simulink model "RobotX_ss_acousticsSingle_Dock_LB_ODOA_1024"  (R2014a)
settings: Solver=FixedStepDiscrete  StartTime=0.0  StopTime=inf  FixedStep=.25  RelTol=1e-3
undefined symbols (not defined in the file): Com1, Com2, Com3, Com4, DiscIntNeverNeededParam, standard
libraries: xpcseriallib x42, simulink x19, slrtlib x7, dspmtrx3 x2, speedgoatlib x2, speedgoatlib_IO102 x1
(part 6 of 7)

== matlab function RobotX_ss_acousticsSingle_Dock_LB_ODOA_1024/Sensors/1024 Comms/Message Selector/HRT Message/MATLAB Function ==
  data: Time input; asciiHRT output; HRTLat input; HRTLong input; HRTMode input; HRTTask input
% This function creates the heartbeat message to be sent from Speedgoat in
% ascii code
% Written by: Edward Zhu
% Date: 9/17/14

function asciiHRT = asciiHRTEncoder(Time, HRTLat, HRTLong, HRTMode, HRTTask)

% Initialize output message vector as the serial output block expects 128
% character message
asciiHRT = uint8(zeros(1,128));

% Convert static strings to ascii code
asciiHRTMsgID = uint8('$RXHRT,');
asciiComma = uint8(',');
asciiDeciPt = uint8('.');
if HRTLat >= 0
    asciiHRTNS = uint8('N,');
else
    HRTLat = -HRTLat;
    asciiHRTNS = uint8('S,');
end
if HRTLong >= 0
    asciiHRTEW = uint8('E,');
else
    HRTLong = -HRTLong;
    asciiHRTEW = uint8('W,');
end
asciiTeamID = uint8('FAUVU,');
asciiMsgEnd = uint8('*');
asciiMsgCRLF = [13 10];

% Convert UTC Time input (hhmmss) into ascii code
asciiTime = uint8(zeros(1,7));
asciiTime(7) = asciiComma;

for timeChar = 1:6
    asciiTime(timeChar) = floor(mod(Time,10^(7-timeChar))/...
        10^(6-timeChar)) + 48;
end

% Convert latitude (dd.mmmmmm) into ascii code
asciiHRTLat = uint8(zeros(1,10));
asciiHRTLat(10) = asciiComma;
asciiHRTLat(3) = asciiDeciPt;

HRTlatInt = floor(HRTLat);
for latIntChar = 1:2
    asciiHRTLat(latIntChar) = floor(mod(HRTlatInt,10^(3-latIntChar))/...
        10^(2-latIntChar)) + 48;
end

HRTlatDeci = mod(HRTLat,HRTlatInt) * 10^6;
for latDeciChar = 1:6
    asciiHRTLat(latDeciChar+3) = floor(mod(HRTlatDeci,10^(7-latDeciChar))/...
        10^(6-latDeciChar)) + 48;
end

% Convert longitude (ddd.mmmmmm) into ascii code
asciiHRTLong = uint8(zeros(1,11));
asciiHRTLong(11) = asciiComma;
asciiHRTLong(4) = asciiDeciPt;

HRTlongInt = floor(HRTLong);
for longIntChar = 1:3
    asciiHRTLong(longIntChar) = floor(mod(HRTlongInt,10^(4-longIntChar))/...
        10^(3-longIntChar)) + 48;
end

HRTlongDeci = mod(HRTLong,HRTlongInt) * 10^6;
for longDeciChar = 1:6
    asciiHRTLong(longDeciChar+4) = floor(mod(HRTlongDeci,10^(7-longDeciChar))/...
        10^(6-longDeciChar)) + 48;
end


% Convert vehicle mode into ascii (1 = RC, 2 = Auto)

% Auto On 
if HRTMode == 3 
    HRTOpMode = 2;
    asciiHRTMode = [uint8(HRTOpMode+48) asciiComma];
else
    HRTOpMode = 1;
    asciiHRTMode = [uint8(HRTOpMode+48) asciiComma];
end

% Convert vehicle task into ascii
HRTTask = HRTTask - 1; % FSM: Init = 1, SSGate = 2, SEA = 3, Dock = 4, LIT = 5, Obst = 6
if HRTTask ~= 1 || 2 || 3 || 4 || 5
    HRTOpTask = 1;
    asciiHRTTask = [uint8(HRTOpTask+48) asciiMsgEnd];
else
    asciiHRTTask = [uint8(HRTTask+48) asciiMsgEnd];
end

% Concat individual ascii arrays into one array
asciiHRTPreChkSum = cat(2,asciiHRTMsgID,asciiTime,asciiHRTLat,asciiHRTNS,asciiHRTLong,asciiHRTEW,...
    asciiTeamID,asciiHRTMode,asciiHRTTask);

% Calculate the checksum of the message from the '$' to the '*' and convert
% to hex
HRTchkSum = uint8(0);

for chksumChar = 1:(length(asciiHRTPreChkSum)-2)
    HRTchkSum = bitxor(HRTchkSum,asciiHRTPreChkSum(chksumChar+1));
end

% Convert the checksum to ascii
HRTchkSum = dec2hex(HRTchkSum);
asciiHRTChkSum = uint8(zeros(1,length(HRTchkSum))+32);
for i = 1:length(HRTchkSum)
    asciiHRTChkSum(i) = uint8(HRTchkSum(i));
end

% Concat the checksum and the '/r/n' to the end of the message
asciiHRTPostChkSum = cat(2,asciiHRTPreChkSum,asciiHRTChkSum,asciiMsgCRLF);

% Output the final message
asciiHRT(1:length(asciiHRTPostChkSum)) = asciiHRTPostChkSum;

== matlab function RobotX_ss_acousticsSingle_Dock_LB_ODOA_1024/Sensors/1024 Comms/Message Selector/HRTLIT Message/MATLAB Function ==
  data: Time input; HRTLat input; HRTLong input; HRTTask input; HRTMode input; LITValid input; asciiHRTLIT output; LITSequence input
function asciiHRTLIT = asciiHRTLITEncoder(Time,HRTLat,HRTLong,HRTTask,HRTMode,LITValid,LITSequence)
% Initialize output message vector as the serial output block expects 128
% character message
asciiHRTLIT = uint8(zeros(1,128));

asciiComma = uint8(',');
asciiDeciPt = uint8('.');
asciiTeamID = uint8('FAUVU,');
asciiMsgEnd = uint8('*');
asciiMsgCRLF = [13 10];

% Convert UTC Time input (hhmmss) into ascii code
asciiTime = uint8(zeros(1,7));
asciiTime(7) = asciiComma;

for timeChar = 1:6
    asciiTime(timeChar) = floor(mod(Time,10^(7-timeChar))/...
        10^(6-timeChar)) + 48;
end

%%%%%%%%%%%%%%%%%%%%%%%%%%%%%%%%%%%%%%%%%%%%%%%%%%%%%%%%%%%%%%%%%%%%
% Heartbeat message
% Convert static strings to ascii code
asciiHRTMsgID = uint8('$RXHRT,');
if HRTLat >= 0
    asciiHRTNS = uint8('N,');
else
    HRTLat = -HRTLat;
    asciiHRTNS = uint8('S,');
end
if HRTLong >= 0
    asciiHRTEW = uint8('E,');
else
    HRTLong = -HRTLong;
    asciiHRTEW = uint8('W,');
end

% Convert latitude (dd.mmmmmm) into ascii code
asciiHRTLat = uint8(zeros(1,10));
asciiHRTLat(10) = asciiComma;
asciiHRTLat(3) = asciiDeciPt;

HRTlatInt = floor(HRTLat);
for latIntChar = 1:2
    asciiHRTLat(latIntChar) = floor(mod(HRTlatInt,10^(3-latIntChar))/...
        10^(2-latIntChar)) + 48;
end

HRTlatDeci = mod(HRTLat,HRTlatInt) * 10^6;
for latDeciChar = 1:6
    asciiHRTLat(latDeciChar+3) = floor(mod(HRTlatDeci,10^(7-latDeciChar))/...
        10^(6-latDeciChar)) + 48;
end

% Convert longitude (ddd.mmmmmm) into ascii code
asciiHRTLong = uint8(zeros(1,11));
asciiHRTLong(11) = asciiComma;
asciiHRTLong(4) = asciiDeciPt;

HRTlongInt = floor(HRTLong);
for longIntChar = 1:3
    asciiHRTLong(longIntChar) = floor(mod(HRTlongInt,10^(4-longIntChar))/...
        10^(3-longIntChar)) + 48;
end

HRTlongDeci = mod(HRTLong,HRTlongInt) * 10^6;
for longDeciChar = 1:6
    asciiHRTLong(longDeciChar+4) = floor(mod(HRTlongDeci,10^(7-longDeciChar))/...
        10^(6-longDeciChar)) + 48;
end

% Convert vehicle mode into ascii (1 = RC, 2 = Auto)

% Auto On 
if HRTMode == 3 
    HRTOpMode = 2;
    asciiHRTMode = [uint8(HRTOpMode+48) asciiComma];
else
    HRTOpMode = 1;
    asciiHRTMode = [uint8(HRTOpMode+48) asciiComma];
end

% Convert vehicle task into ascii
HRTTask = HRTTask - 1; % FSM: Init = 1, SSGate = 2, SEA = 3, Dock = 4, LIT = 5, Obst = 6
if HRTTask ~= 1 || 2 || 3 || 4 || 5
    HRTOpTask = 1;
    asciiHRTTask = [uint8(HRTOpTask+48) asciiMsgEnd];
else
    asciiHRTTask = [uint8(HRTTask+48) asciiMsgEnd];
end

% Concat individual ascii arrays into one array
asciiHRTPreChkSum = cat(2,asciiHRTMsgID,asciiTime,asciiHRTLat,asciiHRTNS,asciiHRTLong,asciiHRTEW,...
    asciiTeamID,asciiHRTMode,asciiHRTTask);

% Calculate the checksum of the message from the '$' to the '*' and convert
% to hex
HRTchkSum = uint8(0);

for chksumChar = 1:(length(asciiHRTPreChkSum)-2)
    HRTchkSum = bitxor(HRTchkSum,asciiHRTPreChkSum(chksumChar+1));
end

% Convert the checksum to ascii
HRTchkSum = dec2hex(HRTchkSum);
asciiHRTChkSum = uint8(zeros(1,length(HRTchkSum))+32);
for i = 1:length(HRTchkSum)
    asciiHRTChkSum(i) = uint8(HRTchkSum(i));
end

% Concat the checksum and the '/r/n' to the end of the message
asciiHRTPostChkSum = cat(2,asciiHRTPreChkSum,asciiHRTChkSum,asciiMsgCRLF);

%%%%%%%%%%%%%%%%%%%%%%%%%%%%%%%%%%%%%%%%%%%%%%%%%%%%%%%%%%%%%%%%%%%%%

% Light tower message
asciiLITMsgID = uint8('$RXLIT,');

% Convert the light sequece into ascii code (1 = R, 2 = B, 3 = G)
asciiLITSeq = uint8(zeros(1,4)+32);
asciiLITSeq(4) = asciiMsgEnd;

if LITValid == 1
    for seqChar = 1:3
        if LITSequence(seqChar) == 1
            LITSequence(seqChar) = uint8('R');
        elseif LITSequence(seqChar) == 2
            LITSequence(seqChar) = uint8('B');
        elseif LITSequence(seqChar) == 3
            LITSequence(seqChar) = uint8('G');
        end
    end
    asciiLITSeq(1:3) = LITSequence;
end

% Concat individual ascii arrays into one array
asciiLITPreChkSum = cat(2,asciiLITMsgID,asciiTime,asciiTeamID,asciiLITSeq);

% Calculate the checksum of the message from the '$' to the '*' and convert
% to hex
LITchkSum = uint8(0);

for chksumChar = 1:(length(asciiLITPreChkSum)-2)
    LITchkSum = bitxor(LITchkSum,asciiLITPreChkSum(chksumChar+1));
end

% Convert the checksum to ascii
LITchkSum = dec2hex(LITchkSum);
asciiLITChkSum = uint8(zeros(1,length(LITchkSum))+32);
for i = 1:length(LITchkSum)
    asciiLITChkSum(i) = uint8(LITchkSum(i));
end

% Concat the checksum and the '/r/n' to the end of the message
asciiLITPostChkSum = cat(2,asciiLITPreChkSum,asciiLITChkSum,asciiMsgCRLF);

%%%%%%%%%%%%%%%%%%%%%%%%%%%%%%%%%%%%%%%%%%%%%%%%%%%%%%%%%%%%%%%%%%%%%%%%%%%

asciiHRTLITPostChkSum = cat(2,asciiHRTPostChkSum,asciiLITPostChkSum);
asciiHRTLIT(1:length(asciiHRTLITPostChkSum)) = asciiHRTLITPostChkSum;

== matlab function RobotX_ss_acousticsSingle_Dock_LB_ODOA_1024/Main FSM/Acoustic Single Point FSM/Report/MATLAB Function ==
  data: X input; Y input; Psi input; Data output
function Data  = Orient(X, Y, Psi)
%Written by Dylan DeGaetano on September 2, 2014
%Last Edited:Dylan DeGaetano on September 10,2014

%This function passes the current pose data added to the angle of the Light 
%buoy This stare forces the Boat to stare at the bouy.This task must be in station 
%keeping mode

persistent holdPose

if isempty(holdPose)
    holdPose = [X, Y, Psi];
end

%Initialize Data variable
Data = zeros(24,1);

%Set desired pose
Data(1) = holdPose(1);
Data(2) = holdPose(2);
Data(3) = holdPose(3);

end

== matlab function RobotX_ss_acousticsSingle_Dock_LB_ODOA_1024/Main FSM/Start//Speedgate/Aim/LLA to NED ==
  data: LLA input; GoalNED output; NED_origin input
function GoalNED = LLA2NEDfun(LLA,NED_origin)
%Written by Anderson Lebbad on September 20, 2014
%Last edited by:
%
%This function converts a target Latitude, Longitude, Altitude (LLA) point
%into North, East, Down (NED) coordinates

%First convert to earth centered, earth fixed frame
GoalECEF = lla2ecef([LLA*(pi/180), 0]');
%Then convert from ECEF to North East Down
GoalNEDvect = ecef2ned(NED_origin'*(pi/180),GoalECEF);
GoalNED = GoalNEDvect(1:2)';


end

function x_ecef = lla2ecef(x_lla)
% LLE2ECEF: Converts from geodetic latitude, longitude, and altitude to earth-centered earth-fixed Cartesian coordinates
% INPUT: latitude phi (rad), longitude lambda (rad), altitude h (m)
% OUTPUT: [x, y, z]' (m) earth-centered earth-fixed Cartesian coordinates
    a = 6378137; % equatorial radius of ellipsoid (semi-major axis) (m)
    b = 6356752; % polar axis radius of ellipsoid (semi-minor axis) (m)

    phi = x_lla(1);
    lambda = x_lla(2);
    h = x_lla(3);
    
    % auxiliar quantities f, e, and N
    f = (a-b)/a;
    e = f*(2-f);
    N = a/sqrt(1-(e*sin(phi))^2);
    x_ecef = [(N+h)*cos(phi)*cos(lambda); (N+h)*cos(phi)*sin(lambda); (N*(1-e^2)+h)*sin(phi)];
end

function [x_ned] = ecef2ned(ned_lla, x_ecef)
% ECEF2NED Converts from earth-centered, earth-fixed Cartesian coordinates to tangent plane
% INPUT:
% 1) x_ecef=[x,y,z]' (m) earth-centered, earth-fixed Cartesian coordinates
% 2) ned_lla=[phi,lambda]' consiting of latitude phi (rad), longitude lambda (rad) of NED origin
% OUTPUT:
% 1) x_ned=[x,y,z]' (m) in NED coordinate system with the origin [phi,lambda]'

    phi = ned_lla(1);
    lambda = ned_lla(2);

    % transformation  matrix
    T = [-sin(phi)*cos(lambda) -sin(phi)*sin(lambda)  cos(phi)
         -sin(lambda)           cos(lambda)           0
          cos(phi)*cos(lambda)   cos(phi)*sin(lambda)  sin(phi)];

     x_ned = T*(x_ecef-lla2ecef([phi, lambda, 0]')); % convert to NED
     x_ned(3) = -x_ned(3);
end

== matlab function RobotX_ss_acousticsSingle_Dock_LB_ODOA_1024/Main FSM/LightTower/Approach Light Tower/GPSMove ==
  data: GoalNED input; X input; Finished output; valid output; Y input; Psi input; pts output
function [Finished,valid,pts] = GPSmove(GoalNED,X,Y,Psi)
%Written by Dylan DeGaetano on September 1, 2014
%Last edited by: Anderson Lebbad
%
%This function will go to a given NED cooridnate, last edit changed the
%goal pt and variable names

persistent Sample
if isempty(Sample)
Sample = 0;
end
Finished = 0;
pts = zeros(8,2);

%If this has been going for a while, reset.
if Sample == 100
    Sample = 0;
end

%If we need to calculate desired points to send, calculate them.
if Sample == 0
    pts(1,1) = X+5*cos(Psi*pi/180);
    pts(1,2) = Y+5*sin(Psi*pi/180);
    pts(8,1) = GoalNED(1,1);
    pts(8,2) = GoalNED(1,2);
    pts(2,:) = pts(1,:) +(1*(GoalNED-pts(1,:))/7);
    pts(3,:) = pts(1,:) +(2*(GoalNED-pts(1,:))/7);
    pts(4,:) = pts(1,:) +(3*(GoalNED-pts(1,:))/7);
    pts(5,:) = pts(1,:) +(4*(GoalNED-pts(1,:))/7);
    pts(6,:) = pts(1,:) +(5*(GoalNED-pts(1,:))/7);
    pts(7,:) = pts(1,:) +(6*(GoalNED-pts(1,:))/7);
    Sample = 1; 
    valid = 1;
    
%If we have already calculated desired points, check if we are within a
%certain range of the desired end point.
else 
    range = sqrt(sum((GoalNED - [X Y]).^2));
    if range <= 5
        Finished = 1;
    end
    valid = 0;
    Sample = Sample + 1;
end

== matlab function RobotX_ss_acousticsSingle_Dock_LB_ODOA_1024/Main FSM/LightTower/Approach Light Tower/MATLAB Function ==
  data: HoldPose output; distance input; ltLoc input; GoalNED output; X input; Y input
function [HoldPose, GoalNED] = fcn(distance, ltLoc, X, Y)
%Written by Michael Benson on October 23, 2014

%This function determines the target NED point for the Sweep Field subtask
%for the Light Tower task.  The target point is Distance meters from the
%current ASV position, and is towards the opposite corner of the subset
%field.

%Find slope between ASV and corner
% slope = (ltLoc(2) - Y)/(ltLoc(1) - X);
% GoalNED = [X - distance*cos(slope), Y - distance*sin(slope)];

pts = zeros(1,2);
desiredHeading = atan2(ltLoc(2)-Y,ltLoc(1)-X);
pts(1,1) = ltLoc(1)+distance*cos(desiredHeading);
pts(1,2) = ltLoc(2)+distance*sin(desiredHeading);
GoalNED = [pts(1,1) pts(1,2)];

holdHeading = atan2(ltLoc(2)-GoalNED(2),ltLoc(1)-GoalNED(1))*180/pi;
HoldPose = [GoalNED, holdHeading];

end

== matlab function RobotX_ss_acousticsSingle_Dock_LB_ODOA_1024/Main FSM/LightTower/Go to Field Corner/CalcTimes ==
  data: pts input; u input; Data output
function Data = calcTimes(pts, u)
%Written by Anderson Lebbad on August 9, 2014
%Last Edited: Dylan DeGaetano September 1, 2014

%Calculates times for the boat to get to points for a trajectory, and
%formats Data for communication

%Initialize
Data = zeros(24,1);
traj = zeros(8,3);
traj(:,1:2) = pts;



for k = 2:8
    %Calculate distance to travel from last point
    distTravel = sqrt(sum((pts(k-1,:)-pts(k,:)).^2));
    %Assume 1m per second speed
    traj(k,3) = traj(k-1,3) + distTravel;
    %Add time based off initial velocity to get to first point past initial
    if k == 2
        traj(k,3) = traj(k,3) + 2.5*abs(2-u);
    end
end


%Output Data
for i=1:8
    for j = 1:3
        Data(3*(i-1)+j) = traj(i,j);
    end
end

== matlab function RobotX_ss_acousticsSingle_Dock_LB_ODOA_1024/Main FSM/Start//Speedgate/Aim/MATLAB Function ==
  data: ssHeldHeading input; ssGateNED input; Data output
function Data  = Orient(ssHeldHeading,ssGateNED)
%Written by Dylan DeGaetano on September 2, 2014
%Last Edited:Dylan DeGaetano on September 10,2014

%This function passes the current pose data added to the angle of the Light 
%buoy This stare forces the Boat to stare at the bouy.This task must be in station 
%keeping mode

persistent holdPose

if isempty(holdPose)
    holdPose = [ssGateNED ssHeldHeading];
end

%Initialize Data variable
Data = zeros(24,1);

%Set desired pose
Data(1) = holdPose(1);
Data(2) = holdPose(2);
Data(3) = holdPose(3);

end

== matlab function RobotX_ss_acousticsSingle_Dock_LB_ODOA_1024/Main FSM/LightTower/Go to Field Corner/GPSMove ==
  data: GoalNED input; X input; Finished output; valid output; Y input; Psi input; pts output
function [Finished,valid,pts] = GPSmove(GoalNED,X,Y,Psi)
%Written by Dylan DeGaetano on September 1, 2014
%Last edited by: Anderson Lebbad
%
%This function will go to a given NED cooridnate, last edit changed the
%goal pt and variable names

% Input of GoalNED is a 10x2 matrix of NED coords where the first row is
% the coord of the docking observation point

persistent Sample
if isempty(Sample)
Sample = 0;
end
Finished = 0;
pts = zeros(8,2);
%$Distance to object in meters
if Sample == 100
    Sample = 0;
end

if Sample == 0
    pts(1,1) = X+5*cos(Psi*pi/180);
    pts(1,2) = Y+5*sin(Psi*pi/180);
    pts(8,1) = GoalNED(1,1);
    pts(8,2) = GoalNED(1,2);
    pts(2,:) = pts(1,:) +(1*(GoalNED(1,:)-pts(1,:))/7);
    pts(3,:) = pts(1,:) +(2*(GoalNED(1,:)-pts(1,:))/7);
    pts(4,:) = pts(1,:) +(3*(GoalNED(1,:)-pts(1,:))/7);
    pts(5,:) = pts(1,:) +(4*(GoalNED(1,:)-pts(1,:))/7);
    pts(6,:) = pts(1,:) +(5*(GoalNED(1,:)-pts(1,:))/7);
    pts(7,:) = pts(1,:) +(6*(GoalNED(1,:)-pts(1,:))/7);
    Sample = 1; 
    valid = 1;
    
else 
    range = sqrt(sum((GoalNED(1,:) - [X Y]).^2));
    if range <= 5
        Finished = 1;
    end
    valid = 0;
    Sample = Sample + 1;
end

== matlab function RobotX_ss_acousticsSingle_Dock_LB_ODOA_1024/Main FSM/Start//Speedgate/Dead Reckon/Calculate Times ==
  data: pts input; u input; Data output
function Data = calcTimes(pts, u)
%Written by Anderson Lebbad on August 9, 2014
%Last Edited:

%Calculates times for the boat to get to points for a trajectory, and
%formats Data for communication

%Initialize
Data = zeros(24,1);
traj = zeros(8,3);

traj(:,1:2) = pts;

for k = 2:8
    %Calculate distance to travel from last point
    distTravel = sqrt(sum((pts(k-1,:)-pts(k,:)).^2));
    %Assume 1m per second speed
    traj(k,3) = traj(k-1,3) + distTravel;
    %Add time based off initial velocity to get to first point past initial
    if k == 2
        traj(k,3) = traj(k,3) + 2.5*abs(2-u);
    end
end


%Output Data
for i=1:8
    for j = 1:3
        Data(3*(i-1)+j) = traj(i,j);
    end
end

== matlab function RobotX_ss_acousticsSingle_Dock_LB_ODOA_1024/Main FSM/Start//Speedgate/Dead Reckon/Gate ==
  data: sglength input; ssHeldHeading input; Finished output; Valid output; X input; Y input; pts output
function [Finished, Valid, pts] = Gate(sglength,ssHeldHeading,X,Y)
%Written by Anderson Lebbad on August 9, 2014
%Last Edited by:

%This function sends a forward trajectory (from the initial heading read
%into it) until a landmark is found. Once the landmark is found, a
%trajectory is written to dodge around it.

pts = zeros(8,2);
Valid = 0;



persistent Found finPt
if isempty(Found)
    Found = 0;
    pts(1,1) = X + 5*cos(ssHeldHeading*pi/180);
    pts(1,2) = Y + 5*sin(ssHeldHeading*pi/180);
    pts(8,1) = X + sglength*cos(ssHeldHeading*pi/180);
    pts(8,2) = Y + sglength*sin(ssHeldHeading*pi/180);
    pts(2:7,:) = (1:6)'*(pts(8,:)-pts(1,:))/7+ones(6,1)*pts(1,:);
    Valid = 1;
    finPt = pts(8,:);
end

Finished = 0;

%Check to see how far the current pose is from the final point in the
%trajectory
range = abs(finPt(1)-X)+abs(finPt(2)-Y);


if range <= 10
    Finished = 1;
end

end

== matlab function RobotX_ss_acousticsSingle_Dock_LB_ODOA_1024/Main FSM/LightTower/Approach Light Tower/CalcTimes ==
  data: pts input; u input; Data output
function Data = calcTimes(pts, u)
%Written by Anderson Lebbad on August 9, 2014
%Last Edited: Dylan DeGaetano September 1, 2014

%Calculates times for the boat to get to points for a trajectory, and
%formats Data for communication

%Initialize
Data = zeros(24,1);
traj = zeros(8,3);
traj(:,1:2) = pts;



for k = 2:8
    %Calculate distance to travel from last point
    distTravel = sqrt(sum((pts(k-1,:)-pts(k,:)).^2));
    %Assume 1m per second speed
    traj(k,3) = traj(k-1,3) + distTravel;
    %Add time based off initial velocity to get to first point past initial
    if k == 2
        traj(k,3) = traj(k,3) + 2.5*abs(2-u);
    end
end


%Output Data
for i=1:8
    for j = 1:3
        Data(3*(i-1)+j) = traj(i,j);
    end
end

== matlab function RobotX_ss_acousticsSingle_Dock_LB_ODOA_1024/Main FSM/Main Enabler ==
  data: taskSelector output; initEn output; startgateEn output; acouEn output; dockEn output; LTEn output; ODOAEn output; termEn output; RCEn output; OnOffRCAuto input; initFin input; startgateFin input; acouFin input; dockFin input; LTFin input; ODOAFin input
function [taskSelector,initEn,startgateEn,acouEn,dockEn,LTEn,ODOAEn,termEn,RCEn] ...
    = taskEnabler(OnOffRCAuto,initFin,startgateFin,acouFin,dockFin,LTFin,ODOAFin)
%Written by Anderson Lebbad on September 13, 2014
%Last Edited by:

%Changes the value of MainMode and the enablers for the tasks within the
%Main FSM.

% Initialize enable signals
RCEn = 0;
initEn = 0;
startgateEn = 0;
termEn = 0;
acouEn = 0;
dockEn = 0;
LTEn = 0;
ODOAEn = 0;

% Set enable signals based on state completion
if initFin == 0
    initEn = 1;
    taskSelector = 1;
elseif OnOffRCAuto ~= 3
    RCEn = 1;
    taskSelector = 8;
elseif startgateFin == 0
    startgateEn = 1;
    taskSelector = 2;
elseif acouFin == 0
    acouEn = 1;
    taskSelector = 3;
elseif dockFin == 0
    dockEn = 1;
    taskSelector = 4;
elseif LTFin == 0
    LTEn = 1;
    taskSelector = 5;
elseif ODOAFin == 0
    ODOAEn = 1;
    taskSelector = 6;
else
    termEn = 1;
    taskSelector = 7;
end

== matlab function RobotX_ss_acousticsSingle_Dock_LB_ODOA_1024/Sensors/1024 Comms/Message Selector/HRTSEA Message/MATLAB Function ==
  data: Time input; HRTLat input; HRTLong input; HRTTask input; HRTMode input; SEAValid input; asciiHRTSEA output; SEALat input; SEALong input; SEAColor input; SEADepth input
function asciiHRTSEA = asciiHRTSEAEncoder(Time,HRTLat,HRTLong,HRTTask,HRTMode,SEAValid,SEALat,SEALong,SEAColor,SEADepth)

% Initialize output message vector as the serial output block expects 128
% character message
asciiHRTSEA = uint8(zeros(1,128));

asciiComma = uint8(',');
asciiDeciPt = uint8('.');
asciiTeamID = uint8('FAUVU,');
asciiMsgEnd = uint8('*');
asciiMsgCRLF = [13 10];

% Convert UTC Time input (hhmmss) into ascii code
asciiTime = uint8(zeros(1,7));
asciiTime(7) = asciiComma;

for timeChar = 1:6
    asciiTime(timeChar) = floor(mod(Time,10^(7-timeChar))/...
        10^(6-timeChar)) + 48;
end

%%%%%%%%%%%%%%%%%%%%%%%%%%%%%%%%%%%%%%%%%%%%%%%%%%%%%%%%%%%%%%%%%%%%
% Heartbeat message
% Convert static strings to ascii code
asciiHRTMsgID = uint8('$RXHRT,');
if HRTLat >= 0
    asciiHRTNS = uint8('N,');
else
    HRTLat = -HRTLat;
    asciiHRTNS = uint8('S,');
end
if HRTLong >= 0
    asciiHRTEW = uint8('E,');
else
    HRTLong = -HRTLong;
    asciiHRTEW = uint8('W,');
end

% Convert latitude (dd.mmmmmm) into ascii code
asciiHRTLat = uint8(zeros(1,10));
asciiHRTLat(10) = asciiComma;
asciiHRTLat(3) = asciiDeciPt;

HRTlatInt = floor(HRTLat);
for latIntChar = 1:2
    asciiHRTLat(latIntChar) = floor(mod(HRTlatInt,10^(3-latIntChar))/...
        10^(2-latIntChar)) + 48;
end

HRTlatDeci = mod(HRTLat,HRTlatInt) * 10^6;
for latDeciChar = 1:6
    asciiHRTLat(latDeciChar+3) = floor(mod(HRTlatDeci,10^(7-latDeciChar))/...
        10^(6-latDeciChar)) + 48;
end

% Convert longitude (ddd.mmmmmm) into ascii code
asciiHRTLong = uint8(zeros(1,11));
asciiHRTLong(11) = asciiComma;
asciiHRTLong(4) = asciiDeciPt;

HRTlongInt = floor(HRTLong);
for longIntChar = 1:3
    asciiHRTLong(longIntChar) = floor(mod(HRTlongInt,10^(4-longIntChar))/...
        10^(3-longIntChar)) + 48;
end

HRTlongDeci = mod(HRTLong,HRTlongInt) * 10^6;
for longDeciChar = 1:6
    asciiHRTLong(longDeciChar+4) = floor(mod(HRTlongDeci,10^(7-longDeciChar))/...
        10^(6-longDeciChar)) + 48;
end

% Convert vehicle mode into ascii (1 = RC, 2 = Auto)

% Auto On 
if HRTMode == 3 
    HRTOpMode = 2;
    asciiHRTMode = [uint8(HRTOpMode+48) asciiComma];
else
    HRTOpMode = 1;
    asciiHRTMode = [uint8(HRTOpMode+48) asciiComma];
end

% Convert vehicle task into ascii
HRTTask = HRTTask - 1; % FSM: Init = 1, SSGate = 2, SEA = 3, Dock = 4, LIT = 5, Obst = 6
if HRTTask ~= 1 || 2 || 3 || 4 || 5
    HRTOpTask = 1;
    asciiHRTTask = [uint8(HRTOpTask+48) asciiMsgEnd];
else
    asciiHRTTask = [uint8(HRTTask+48) asciiMsgEnd];
end

% Concat individual ascii arrays into one array
asciiHRTPreChkSum = cat(2,asciiHRTMsgID,asciiTime,asciiHRTLat,asciiHRTNS,asciiHRTLong,asciiHRTEW,...
    asciiTeamID,asciiHRTMode,asciiHRTTask);

% Calculate the checksum of the message from the '$' to the '*' and convert
% to hex
HRTchkSum = uint8(0);

for chksumChar = 1:(length(asciiHRTPreChkSum)-2)
    HRTchkSum = bitxor(HRTchkSum,asciiHRTPreChkSum(chksumChar+1));
end

% Convert the checksum to ascii
HRTchkSum = dec2hex(HRTchkSum);
asciiHRTChkSum = uint8(zeros(1,length(HRTchkSum))+32);
for i = 1:length(HRTchkSum)
    asciiHRTChkSum(i) = uint8(HRTchkSum(i));
end

% Concat the checksum and the '/r/n' to the end of the message
asciiHRTPostChkSum = cat(2,asciiHRTPreChkSum,asciiHRTChkSum,asciiMsgCRLF);

%%%%%%%%%%%%%%%%%%%%%%%%%%%%%%%%%%%%%%%%%%%%%%%%%%%%%%%%%%%%%%%%%%%%%

% Underwater search message
asciiSEAMsgID = uint8('$RXSEA,');
if SEAValid == 1
    if SEALat >= 0
        asciiSEANS = uint8('N,');
    else
        SEALat = -SEALat;
        asciiSEANS = uint8('S,');
    end
    if SEALong >= 0
        asciiSEAEW = uint8('E,');
    else
        SEALong = -SEALong;
        asciiSEAEW = uint8('W,');
    end
else
    asciiSEANS = [32 asciiComma];
    asciiSEAEW = [32 asciiComma];
end

% Convert buoy color to ascii code (1 = R, 2 = G, 3 = B, 4 = W, 5 = K)
asciiSEAColor = [uint8(32) asciiComma]; % Initialize as whitespace in case no buoy is found

if SEAColor == 1
    asciiSEAColor(1) = uint8('R');
elseif SEAColor == 2
    asciiSEAColor(1) = uint8('G');
elseif SEAColor == 3
    asciiSEAColor(1) = uint8('B');
elseif SEAColor == 4
    asciiSEAColor(1) = uint8('W');
elseif SEAColor == 5
    asciiSEAColor(1) = uint8('K');
end

% Convert latitude (dd.mmmmmm) into ascii code
asciiSEALat = uint8(zeros(1,10)+32); % Initialize as whitespace in case no buoy is found
asciiSEALat(10) = asciiComma;

% Only output values if valid bit is high
if SEAValid == 1
    asciiSEALat(3) = asciiDeciPt;
    SEAlatInt = floor(SEALat);
    for latIntChar = 1:2
        asciiSEALat(latIntChar) = floor(mod(SEAlatInt,10^(3-latIntChar))/...
            10^(2-latIntChar)) + 48;
    end
    
    SEAlatDeci = mod(SEALat,SEAlatInt) * 10^6;
    for latDeciChar = 1:6
        asciiSEALat(latDeciChar+3) = floor(mod(SEAlatDeci,10^(7-latDeciChar))/...
            10^(6-latDeciChar)) + 48;
    end
end

% Convert longitude (ddd.mmmmmm) into ascii code
asciiSEALong = uint8(zeros(1,11)+32); % Initialize as whitespace in case no buoy is found
asciiSEALong(11) = asciiComma;

% Only output values if valid bit is high
if SEAValid == 1
    asciiSEALong(4) = asciiDeciPt;
    SEAlongInt = floor(SEALong);
    for longIntChar = 1:3
        asciiSEALong(longIntChar) = floor(mod(SEAlongInt,10^(4-longIntChar))/...
            10^(3-longIntChar)) + 48;
    end
    
    SEAlongDeci = mod(SEALong,SEAlongInt) * 10^6;
    for longDeciChar = 1:6
        asciiSEALong(longDeciChar+4) = floor(mod(SEAlongDeci,10^(7-longDeciChar))/...
            10^(6-longDeciChar)) + 48;
    end
end

% Convert depth (m) (##.##) into ascii
asciiSEADepth = uint8(zeros(1,6)+32); % Initialize as whitespace in case no buoy is found
asciiSEADepth(6) = asciiMsgEnd;

% Only output values if valid bit is high
if SEAValid == 1
    asciiSEADepth(3) = asciiDeciPt;
    SEAdepthInt = floor(SEADepth);
    for depthIntChar = 1:2
        asciiSEADepth(depthIntChar) = floor(mod(SEAdepthInt,10^(3-depthIntChar))/...
            10^(2-depthIntChar)) + 48;
    end
    
    SEAdepthDeci = mod(SEADepth,SEAdepthInt) * 10^2;
    for depthDeciChar = 1:2
        asciiSEADepth(depthDeciChar+3) = floor(mod(SEAdepthDeci,10^(3-depthDeciChar))/...
            10^(2-depthDeciChar)) + 48;
    end
end

% Concat individual ascii arrays into one array
asciiSEAPreChkSum = cat(2,asciiSEAMsgID,asciiTime,asciiTeamID,asciiSEAColor,...
    asciiSEALat,asciiSEANS,asciiSEALong,asciiSEAEW,asciiSEADepth);

% Calculate the checksum of the message from the '$' to the '*' and convert
% to hex
SEAchkSum = uint8(0);

for chksumChar = 1:(length(asciiSEAPreChkSum)-2)
    SEAchkSum = bitxor(SEAchkSum,asciiSEAPreChkSum(chksumChar+1));
end

% Convert the checksum to ascii
SEAchkSum = dec2hex(SEAchkSum);
asciiSEAChkSum = uint8(zeros(1,length(SEAchkSum))+32);
for i = 1:length(SEAchkSum)
    asciiSEAChkSum(i) = uint8(SEAchkSum(i));
end

% Concat the checksum and the '/r/n' to the end of the message
asciiSEAPostChkSum = cat(2,asciiSEAPreChkSum,asciiSEAChkSum,asciiMsgCRLF);

%%%%%%%%%%%%%%%%%%%%%%%%%%%%%%%%%%%%%%%%%%%%%%%%%%%%%%%%%%%%%%%%%%%%%%

asciiHRTSEAPostChkSum = cat(2,asciiHRTPostChkSum,asciiSEAPostChkSum);
asciiHRTSEA(1:length(asciiHRTSEAPostChkSum)) = asciiHRTSEAPostChkSum;

== matlab function RobotX_ss_acousticsSingle_Dock_LB_ODOA_1024/Main FSM/Start//Speedgate/GPS Move/CalcTimes ==
  data: pts input; u input; Data output
function Data = calcTimes(pts, u)
%Written by Anderson Lebbad on August 9, 2014
%Last Edited: Dylan DeGaetano September 1, 2014

%Calculates times for the boat to get to points for a trajectory, and
%formats Data for communication

%Initialize
Data = zeros(24,1);
traj = zeros(8,3);
traj(:,1:2) = pts;



for k = 2:8
    %Calculate distance to travel from last point
    distTravel = sqrt(sum((pts(k-1,:)-pts(k,:)).^2));
    %Assume 1m per second speed
    traj(k,3) = traj(k-1,3) + distTravel;
    %Add time based off initial velocity to get to first point past initial
    if k == 2
        traj(k,3) = traj(k,3) + 2.5*abs(2-u);
    end
end


%Output Data
for i=1:8
    for j = 1:3
        Data(3*(i-1)+j) = traj(i,j);
    end
end

== matlab function RobotX_ss_acousticsSingle_Dock_LB_ODOA_1024/Main FSM/Start//Speedgate/GPS Move/LLA to NED ==
  data: LLA input; GoalNED output; NED_origin input
function GoalNED = LLA2NEDfun(LLA,NED_origin)
%Written by Anderson Lebbad on September 20, 2014
%Last edited by:
%
%This function converts a target Latitude, Longitude, Altitude (LLA) point
%into North, East, Down (NED) coordinates

%First convert to earth centered, earth fixed frame
GoalECEF = lla2ecef([LLA*(pi/180), 0]');
%Then convert from ECEF to North East Down
GoalNEDvect = ecef2ned(NED_origin'*(pi/180),GoalECEF);
GoalNED = GoalNEDvect(1:2)';


end

function x_ecef = lla2ecef(x_lla)
% LLE2ECEF: Converts from geodetic latitude, longitude, and altitude to earth-centered earth-fixed Cartesian coordinates
% INPUT: latitude phi (rad), longitude lambda (rad), altitude h (m)
% OUTPUT: [x, y, z]' (m) earth-centered earth-fixed Cartesian coordinates
    a = 6378137; % equatorial radius of ellipsoid (semi-major axis) (m)
    b = 6356752; % polar axis radius of ellipsoid (semi-minor axis) (m)

    phi = x_lla(1);
    lambda = x_lla(2);
    h = x_lla(3);
    
    % auxiliar quantities f, e, and N
    f = (a-b)/a;
    e = f*(2-f);
    N = a/sqrt(1-(e*sin(phi))^2);
    x_ecef = [(N+h)*cos(phi)*cos(lambda); (N+h)*cos(phi)*sin(lambda); (N*(1-e^2)+h)*sin(phi)];
end

function [x_ned] = ecef2ned(ned_lla, x_ecef)
% ECEF2NED Converts from earth-centered, earth-fixed Cartesian coordinates to tangent plane
% INPUT:
% 1) x_ecef=[x,y,z]' (m) earth-centered, earth-fixed Cartesian coordinates
% 2) ned_lla=[phi,lambda]' consiting of latitude phi (rad), longitude lambda (rad) of NED origin
% OUTPUT:
% 1) x_ned=[x,y,z]' (m) in NED coordinate system with the origin [phi,lambda]'

    phi = ned_lla(1);
    lambda = ned_lla(2);

    % transformation  matrix
    T = [-sin(phi)*cos(lambda) -sin(phi)*sin(lambda)  cos(phi)
         -sin(lambda)           cos(lambda)           0
          cos(phi)*cos(lambda)   cos(phi)*sin(lambda)  sin(phi)];

     x_ned = T*(x_ecef-lla2ecef([phi, lambda, 0]')); % convert to NED
     x_ned(3) = -x_ned(3);
end

== matlab function RobotX_ss_acousticsSingle_Dock_LB_ODOA_1024/Main FSM/LightTower/Point Toward Last Known Heading/Look for Light Tower ==
  data: SubBox input; X input; Y input; Psi input; Distances input; Angles input; lastKnownNED input; Data output; Finished output; FoundTower output; TowerLoc output
function [Data, Finished, FoundTower, TowerLoc] = lightTowerSearch(...
    SubBox, X, Y, Psi, Distances, Angles, lastKnownNED)

%   Written by Michael Benson on October 23, 2014
%   This function looks for the light tower after being pointed at the last
%   known heading to the light tower by the previous task.  If the Lidar
%   sees an object, and that object is within the field subset, the boat
%   will hold pose and the Lidar will continue to evaluate an object.  If
%   the object is still there within that time, it determines that that
%   object is the buoy and ends the task.  Otherwise, the task exits
%   without setting FoundTower high.

[Distances,I] = sort(Distances);
Angles = Angles(I);
Psi = Psi*180/pi;

persistent notFoundCounter desiredHeading

if isempty(desiredHeading) && isempty(notFoundCounter)
    notFoundCounter = 0;
    desiredHeading = mod(atan2(lastKnownNED(2)-Y,lastKnownNED(1)-X)*180/pi+360,360);
end

Finished = 0;
FoundTower = 0;
Data = zeros(24,1);
Data(1:3) = [X Y desiredHeading];
TowerLoc = zeros(1,2);
tmpGoal = zeros(1,2);
LandmarkLocations = zeros(12,2);
LandmarkDistances = zeros(12,1);

ObjectInfo = [Distances Angles];
diffHeading = Psi - desiredHeading;

if abs(diffHeading) < 5
    %If no objects are found, increment not Found counter
    if ObjectInfo(12,1) == 0 && ObjectInfo(12,2) == 0
        notFoundCounter = notFoundCounter + 1;
    else
        %calculate location of each landmark and determine if it is in the
        %bounding box
        for i = 12-sum(Distances ~= 0)+1:12
            LandmarkX = X + cos(Psi+Angles(i))*Distances(i)/100;
            LandmarkY = Y + sin(Psi+Angles(i))*Distances(i)/100;
            LandmarkValid = inBbox(SubBox,[LandmarkX, LandmarkY]);
            if LandmarkValid == 1
                LandmarkLocations(i,1:2) = [LandmarkX, LandmarkY];
                LandmarkDistances(i) = Distances(i);
            end
        end
        notFoundCounter = 0;
        
        [~,I] = sort(LandmarkDistances);
        LandmarkLocations = LandmarkLocations(I);
        
        if sum(LandmarkDistances ~= 0) >= 1
            tmpGoal = LandmarkLocations(12-sum(LandmarkDistances ~= 0)+1,1:2);
            TowerLoc = tmpGoal;
            FoundTower = 1;
            notFoundCounter = 0;
        else
            notFoundCounter = notFoundCounter + 1;
        end
    end
    
    if notFoundCounter >= 40
        Finished = 1;
    end
end

end
%     %If we have looked at the object for 2 seconds and it is still valid, it's
%     %the light tower
%     if FoundCounter == 8 && evaluating == 1 && idx ~= 0
%         Finished = 1;
%         FoundTower = 1;
%
%         %If we have looked at the object for less than 2 seconds, but think it's
%         %good, check if it's moved far.  If it's moved very far, stop evaluating.
%     elseif FoundCounter < 8 && FoundCounter > 1 && evaluating == 1 && idx ~= 0
%         AngleChange = abs(lastAngle - Angles(idx));
%         DistanceChange = abs(lastDistance - Distances(idx));
%         if AngleChange > 10 || DistanceChange > 500
%             evaluating = 0;
%             Finished = 1;
%             TowerLoc = [X + Distances(idx)*cosd(Psi+Angles(idx)),...
%                 Y+Distances(idx)*sind(Psi+Angles(idx))];
%         end
%     end
%
%     lastAngle = Angles(idx);
%     lastDistance = Distances(idx);

function [ inBbox ] = inBbox( bbox, point )
%UNTITLED Summary of this function goes here
%   Detailed explanation goes here
b1 = bbox(1,:);
b2 = bbox(2,:);
b3 = bbox(3,:);
b4 = bbox(4,:);

t1 = inTriangle(point,b1,b2,b3);
t2 = inTriangle(point,b1,b2,b4);
t3 = inTriangle(point,b1,b3,b4);

if t1 && t2 && t3
    inBbox = 1;
else
    inBbox = 0;
end

end

function [ inTri ] = inTriangle(p, a, b, c)

s1 = sameSide(p,a,b,c);
s2 = sameSide(p,b,a,c);
s3 = sameSide(p,c,a,b);

if s1 || s2 || s3
    inTri = 1;
else
    inTri = 0;
end

end

function [ onSame ] = sameSide(p1,p2,a,b)

theta = atan2(b(2)-a(2),b(1)-a(1));
R = [cos(theta), sin(theta); -sin(theta), cos(theta)];
side1 = R*(p1-a)';
side2 = R*(p2-a)';
same = side1(2)/side2(2);
onSame = same >= 0;

end

== matlab function RobotX_ss_acousticsSingle_Dock_LB_ODOA_1024/Sensors/1020 Comms/MATLAB Function1 ==
  data: Valid input; Time input; asciiSEA output; Lat input; Long input; Color input; Depth input
% This function creates the underwater search message to be sent from 
% Speedgoat in ascii code
% Written by: Edward Zhu
% Date: 9/17/14

function asciiSEA = asciiSEAEncoder(Valid, Time, Lat, Long, Color, Depth)

% Initialize output message vector as the serial output block expects 128
% character message
asciiSEA = uint8(zeros(1,128));

% Convert static strings to ascii code
asciiMsgID = uint8('$RXSEA,');
asciiComma = uint8(',');
asciiDeciPt = uint8('.');
if Valid == 1
    if Lat >= 0
        asciiNS = uint8('N,');
    else
        Lat = -Lat;
        asciiNS = uint8('S,');
    end
    if Long >= 0
        asciiEW = uint8('E,');
    else
        Long = -Long;
        asciiEW = uint8('W,');
    end
else
    asciiNS = [32 asciiComma];
    asciiEW = [32 asciiComma];
end
asciiTeamID = uint8('FAUVU,');
asciiMsgEnd = uint8('*');
asciiMsgCRLF = [13 10];

% Convert UTC Time input (hhmmss) into ascii code
asciiTime = uint8(zeros(1,7));
asciiTime(7) = asciiComma;

for timeChar = 1:6
    asciiTime(timeChar) = floor(mod(Time,10^(7-timeChar))/...
        10^(6-timeChar)) + 48;
end

% Convert buoy color to ascii code (1 = R, 2 = G, 3 = B, 4 = W, 5 = K)
asciiColor = [uint8(32) asciiComma]; % Initialize as whitespace in case no buoy is found
if Valid == 1
    if Color == 1
        asciiColor(1) = uint8('R');
    elseif Color == 2
        asciiColor(1) = uint8('G');
    elseif Color == 3
        asciiColor(1) = uint8('B');
    elseif Color == 4
        asciiColor(1) = uint8('W');
    elseif Color == 5
        asciiColor(1) = uint8('K');
    end
end
% Convert latitude (dd.mmmmmm) into ascii code
asciiLat = uint8(zeros(1,10)+32); % Initialize as whitespace in case no buoy is found
asciiLat(10) = asciiComma;

% Only output values if valid bit is high
if Valid == 1
    asciiLat(3) = asciiDeciPt;
    latInt = floor(Lat);
    for latIntChar = 1:2
        asciiLat(latIntChar) = floor(mod(latInt,10^(3-latIntChar))/...
            10^(2-latIntChar)) + 48;
    end
    
    latDeci = mod(Lat,latInt) * 10^6;
    for latDeciChar = 1:6
        asciiLat(latDeciChar+3) = floor(mod(latDeci,10^(7-latDeciChar))/...
            10^(6-latDeciChar)) + 48;
    end
end

% Convert longitude (ddd.mmmmmm) into ascii code
asciiLong = uint8(zeros(1,11)+32); % Initialize as whitespace in case no buoy is found
asciiLong(11) = asciiComma;

% Only output values if valid bit is high
if Valid == 1
    asciiLong(4) = asciiDeciPt;
    longInt = floor(Long);
    for longIntChar = 1:3
        asciiLong(longIntChar) = floor(mod(longInt,10^(4-longIntChar))/...
            10^(3-longIntChar)) + 48;
    end
    
    longDeci = mod(Long,longInt) * 10^6;
    for longDeciChar = 1:6
        asciiLong(longDeciChar+4) = floor(mod(longDeci,10^(7-longDeciChar))/...
            10^(6-longDeciChar)) + 48;
    end
end

% Convert depth (m) (##.##) into ascii
asciiDepth = uint8(zeros(1,6)+32); % Initialize as whitespace in case no buoy is found
asciiDepth(6) = asciiMsgEnd;

% Only output values if valid bit is high
if Valid == 1
    asciiDepth(3) = asciiDeciPt;
    depthInt = floor(Depth);
    for depthIntChar = 1:2
        asciiDepth(depthIntChar) = floor(mod(depthInt,10^(3-depthIntChar))/...
            10^(2-depthIntChar)) + 48;
    end
    
    depthDeci = mod(Depth,depthInt) * 10^2;
    for depthDeciChar = 1:2
        asciiDepth(depthDeciChar+3) = floor(mod(depthDeci,10^(3-depthDeciChar))/...
            10^(2-depthDeciChar)) + 48;
    end
end

% Concat individual ascii arrays into one array
asciiPreChkSum = cat(2,asciiMsgID,asciiTime,asciiTeamID,asciiColor,...
    asciiLat,asciiNS,asciiLong,asciiEW,asciiDepth);

% Calculate the checksum of the message from the '$' to the '*' and convert
% to hex
chkSum = uint8(0);

for chksumChar = 1:(length(asciiPreChkSum)-2)
    chkSum = bitxor(chkSum,asciiPreChkSum(chksumChar+1));
end

% Convert the checksum to ascii
chkSum = dec2hex(chkSum);
asciiChkSum = uint8(zeros(1,length(chkSum))+32);
for i = 1:length(chkSum)
    asciiChkSum(i) = uint8(chkSum(i));
end

% Concat the checksum and the '/r/n' to the end of the message
asciiPostChkSum = cat(2,asciiPreChkSum,asciiChkSum,asciiMsgCRLF);

% Output the final message
asciiSEA(1:length(asciiPostChkSum)) = asciiPostChkSum;

== matlab function RobotX_ss_acousticsSingle_Dock_LB_ODOA_1024/Main FSM/LightTower/Sweep Field/Drive to Point/MATLAB Function ==
  data: X input; Y input; Psi input; dist input; GoalNED output
function GoalNED = fcn(X, Y, Psi, dist)
%Written by Michael Benson on October 23, 2014

%This function determines the target NED point for the Sweep Field subtask
%for the Light Tower task.  The target point is Distance meters from the
%current ASV position, and is towards the opposite corner of the subset
%field.
pts = zeros(1,2);

%Find slope between ASV and corner
pts(1,1) = X+dist*cos(Psi*pi/180);
pts(1,2) = Y+dist*sin(Psi*pi/180);
GoalNED = [pts(1,1) pts(1,2)];

== matlab function RobotX_ss_acousticsSingle_Dock_LB_ODOA_1024/Main FSM/LightTower/Report and Manuever Away/CalcTimes ==
  data: pts input; u input; Data output
function Data = calcTimes(pts, u)
%Written by Anderson Lebbad on August 9, 2014
%Last Edited: Dylan DeGaetano September 1, 2014

%Calculates times for the boat to get to points for a trajectory, and
%formats Data for communication

%Initialize
Data = zeros(24,1);
traj = zeros(8,3);
traj(:,1:2) = pts;



for k = 2:8
    %Calculate distance to travel from last point
    distTravel = sqrt(sum((pts(k-1,:)-pts(k,:)).^2));
    %Assume 1m per second speed
    traj(k,3) = traj(k-1,3) + distTravel;
    %Add time based off initial velocity to get to first point past initial
    if k == 2
        traj(k,3) = traj(k,3) + 2.5*abs(2-u);
    end
end


%Output Data
for i=1:8
    for j = 1:3
        Data(3*(i-1)+j) = traj(i,j);
    end
end

== matlab function RobotX_ss_acousticsSingle_Dock_LB_ODOA_1024/Main FSM/LightTower/Point Toward Last Known Heading/Light Tower Field Subset Corners1 ==
  data: Distance input; givenCorners input; SubBox output
function SubBox = FieldSubsetCorners(Distance, givenCorners)

%Written by Michael Benson on October 23, 2014

%This function takes in the given NED field corners for the light tower
%task, and a desired distance, and returns a subset of that field with
%corners Distance meters away from the original respective corners.

% Assumes that the subset corners are given in a clockwise manner, ex: 
% 1 - topLeft
% 2 - topRight
% 3 - bottomLeft
% 4 - bottomRight

% The first corner needs to be the corner closest to where the boat should
% go if it does not find the light tower in this subtask, i.e. the corner
% closest to the dock.

SubBox = zeros(4,2);

SubBox(1,:) = [givenCorners(1,1)-Distance givenCorners(1,2)+Distance];
SubBox(2,:) = [givenCorners(2,1)-Distance givenCorners(2,2)-Distance];
SubBox(3,:) = [givenCorners(3,1)+Distance givenCorners(3,2)+Distance];
SubBox(4,:) = [givenCorners(4,1)+Distance givenCorners(4,2)-Distance];

== matlab function RobotX_ss_acousticsSingle_Dock_LB_ODOA_1024/Main FSM/LightTower/Sweep Field/Task Option/Message Composer ==
  data: taskStrInit input; taskStrAdj output
function taskStrAdj = composeMessage(taskStrInit)
%Written by Anderson Lebbad on August 9, 2013
%Last Edited: Edward Zhu on June 2, 2014

%This function adjusts the length of a vector to a set value by filling
%the remaining space with 0's. This is necessary for data store objects
%that have a fixed size for the memory allocation, but a variable length
%input.

%Length of message packet
strLength = 8;

%Size of text in message
taskStrLength = size(taskStrInit,1);

%Pad end of text with zeros
taskStrAdj = [taskStrInit' zeros(1,strLength-taskStrLength)];

== matlab function RobotX_ss_acousticsSingle_Dock_LB_ODOA_1024/Main FSM/LightTower/Turn For Approach1 /MATLAB1 Function ==
  data: LTLoc input; X input; Data output; Y input
function Data  = Orient1(LTLoc, X, Y)
%Written by Dylan DeGaetano on September 2, 2014
%Last Edited:Dylan DeGaetano on September 10,2014

%This function passes the current pose data added to the angle of the Light 
%buoy This stare forces the Boat to stare at the bouy.This task must be in station 
%keeping mode

persistent holdPose

desiredHeading = mod(atan2(LTLoc(2)-Y,LTLoc(1)-X)*180/pi,360);

if isempty(holdPose)
    holdPose = [X, Y, desiredHeading];
end

%Initialize Data variable
Data = zeros(24,1);

%Set desired pose
Data(1) = holdPose(1);
Data(2) = holdPose(2);
Data(3) = holdPose(3);

end

== matlab function RobotX_ss_acousticsSingle_Dock_LB_ODOA_1024/Main FSM/ODOA/Entry Gate/Entry Gate Align/MATLAB Function1 ==
  data: EnterGateNED input; entryNED output; gateNumber input
function entryNED = EntryGPSSelector(EnterGateNED,gateNumber)

entryNED = EnterGateNED(gateNumber,:);

== matlab function RobotX_ss_acousticsSingle_Dock_LB_ODOA_1024/Main FSM/ODOA/Entry Gate/Entry Gate Enabler ==
  data: StartFin input; TaskSelector output; StartEn output; AlignFin input; AlignEn output; ThroughEn output
function [TaskSelector, StartEn,AlignEn,ThroughEn] = entryGateEnabler(StartFin, AlignFin)

StartEn = 0;
AlignEn = 0;
ThroughEn = 0;

if StartFin == 0
    StartEn = 1;
    TaskSelector = 1;
elseif AlignFin == 0
    AlignEn = 1;
    TaskSelector = 2;
else
    ThroughEn = 1;
    TaskSelector = 3;
end

== matlab function RobotX_ss_acousticsSingle_Dock_LB_ODOA_1024/Main FSM/ODOA/Entry Gate/Entry Gate Through/CalcTimes ==
  data: pts input; u input; Data output
function Data = calcTimes(pts, u)
%Written by Anderson Lebbad on August 9, 2014
%Last Edited: Dylan DeGaetano September 1, 2014

%Calculates times for the boat to get to points for a trajectory, and
%formats Data for communication

%Initialize
Data = zeros(24,1);
traj = zeros(8,3);
traj(:,1:2) = pts;



for k = 2:8
    %Calculate distance to travel from last point
    distTravel = sqrt(sum((pts(k-1,:)-pts(k,:)).^2));
    %Assume 1m per second speed
    traj(k,3) = traj(k-1,3) + distTravel;
    %Add time based off initial velocity to get to first point past initial
    if k == 2
        traj(k,3) = traj(k,3) + 2.5*abs(2-u);
    end
end


%Output Data
for i=1:8
    for j = 1:3
        Data(3*(i-1)+j) = traj(i,j);
    end
end

== matlab function RobotX_ss_acousticsSingle_Dock_LB_ODOA_1024/Main FSM/ODOA/Entry Gate/GPS Move/CalcTimes ==
  data: pts input; u input; Data output
function Data = calcTimes(pts, u)
%Written by Anderson Lebbad on August 9, 2014
%Last Edited: Dylan DeGaetano September 1, 2014

%Calculates times for the boat to get to points for a trajectory, and
%formats Data for communication

%Initialize
Data = zeros(24,1);
traj = zeros(8,3);
traj(:,1:2) = pts;



for k = 2:8
    %Calculate distance to travel from last point
    distTravel = sqrt(sum((pts(k-1,:)-pts(k,:)).^2));
    %Assume 1m per second speed
    traj(k,3) = traj(k-1,3) + distTravel;
    %Add time based off initial velocity to get to first point past initial
    if k == 2
        traj(k,3) = traj(k,3) + 2.5*abs(2-u);
    end
end


%Output Data
for i=1:8
    for j = 1:3
        Data(3*(i-1)+j) = traj(i,j);
    end
end

== matlab function RobotX_ss_acousticsSingle_Dock_LB_ODOA_1024/Main FSM/ODOA/Exit Gate/Exit Gate Align/MATLAB Function ==
  data: QuayHeading input; Time input; Data output; X input; Y input; Psi input; Distances input; Angles input; Finished output
function [Data, Finished] = EnterGate(QuayHeading, Time, X, Y, Psi, Distances, Angles)

persistent counter desiredHeading holdPose pos holdTime initPose minPose maxPose minReached maxReached

offset = 5;
spinAmount = 30;

if isempty(counter) && isempty(desiredHeading) && isempty(holdPose) && isempty(pos) && isempty(initPose) && isempty(minReached) && isempty(maxReached) && isempty(minPose) && isempty(maxPose)
    counter = 0;
    holdPose = [X Y mod(QuayHeading+180,360)];
    pos = 0;
    holdTime = Time;
    initPose = [X Y Psi];
    minPose = Psi - spinAmount/2;
    maxPose = Psi + spinAmount/2;
    minReached = 0;
    maxReached = 0;
    desiredHeading = Psi+offset;
end

Finished = 0;
DistM = Distances/100;

[DistM,I] = sort(DistM);
Angles = Angles(I);
ObjectInfo = [DistM Angles];
Data = zeros(24,1);

range = sqrt(sum([initPose(1)-X initPose(2)-Y].^2));

if range < 2 && Time-holdTime > 5
    if sum(DistM ~= 0) <= 1
        if abs(Psi-maxPose) < 5
            maxReached = 1;
        elseif abs(Psi-minPose) < 5
            minReached = 1;
        end
        
        if maxReached == 1
            desiredHeading = Psi - offset;
        elseif maxReached == 1 && minReached == 1
            desiredHeading = initPose(3);
        end
        
        holdPose = [initPose(1:2) desiredHeading];
    else
        closest2Obj = ObjectInfo(12-sum(DistM ~= 0)+1:12-sum(DistM ~= 0)+2,:);
        aveHeading = sum(closest2Obj(:,2))/2;
        desiredHeading = aveHeading + Psi;
        holdPose = [initPose(1:2) desiredHeading];
        counter = counter + 1;
        if counter >= 20
            Finished = 1;
        end
    end
end

Data(1:3) = holdPose;

== matlab function RobotX_ss_acousticsSingle_Dock_LB_ODOA_1024/Main FSM/ODOA/Exit Gate/exit Gate Enabler ==
  data: TaskSelector output; AlignFin input; AlignEn output; ThroughEn output
function [TaskSelector, AlignEn,ThroughEn] = exitGateEnabler(AlignFin)

AlignEn = 0;
ThroughEn = 0;

if AlignFin == 0
    AlignEn = 1;
    TaskSelector = 1;
else
    ThroughEn = 1;
    TaskSelector = 1;
end
